simulink model "siasun_config_casadi_VS_lsj_sim_16a"  (R2020a)
(part 10 of 11)

-0.644078158142065,-0.644802838030618,-0.645527980509147,-0.646253539045693,-0.646979466239331,-0.647705713820167,-0.648432232649345,-0.649158972719038,-0.649885883152457,-0.650612912203845,-0.651340007258479,-0.652067114832670,-0.652794180573764,-0.653521149260139,-0.654247964801207,-0.654974570237416,-0.655700907740245,-0.656426918612209,-0.657152543286855,-0.657877721328767,-0.658602391433560,-0.659326491427883,-0.660049958269421,-0.660772728046890,-0.661494735980042,-0.662215916419663,-0.662936202847570,-0.663655527876618,-0.664373823250693,-0.665091019844716,-0.665807047664642,-0.666521835847457,-0.667235312661186,-0.667947405504885,-0.668658040908642,-0.669367144533582,-0.670074641171864,-0.670780454746678,-0.671484508312250,-0.672186724053839,-0.672887023287738,-0.673585326461276,-0.674281553152812,-0.674975622072357,-0.675667451285948,-0.676356959326780,-0.677044065777502,-0.677728691290112,-0.678410757585964,-0.679090187455765,-0.679766904759571,-0.680440834426794,-0.681111902456198,-0.681780035915898,-0.682445162943365,-0.683107212745418,-0.683766115598233,-0.684421802847337,-0.685074206907609,-0.685723261263280,-0.686368900467938,-0.687011060144518,-0.687649676985311,-0.688284688751960,-0.688916034275461,-0.689543653456161,-0.690167487263763,-0.690787477737318,-0.691403567985234,-0.692015702185270,-0.692623825584536,-0.693227884499498,-0.693827826315972,-0.694423599489128,-0.695015153543487,-0.695602439072925,-0.696185407740670,-0.696764012279302,-0.697338206490753,-0.697907945246309,-0.698473184486608,-0.699033881221643,-0.699589993530754,-0.700141480562639,-0.700688302535347,-0.701230420736280,-0.701767797522191,-0.702300396319188,-0.702828181622730,-0.703351118997629,-0.703869175078051,-0.704382317567512,-0.704890515238883,-0.705393737934386,-0.705891956565598,-0.706385143113447,-0.706873270628213,-0.707356313229530,-0.707834246106384,-0.708307045517114,-0.708774688789411,-0.709237154320320,-0.709694421576238,-0.710146471092914,-0.710593284475450,-0.711034844398302,-0.711471134605276,-0.711902139909533,-0.712327846193585,-0.712748240409299,-0.713163310577893,-0.713573045789936,-0.713977436205353,-0.714376473053420,-0.714770148632767,-0.715158456311373,-0.715541390526574,-0.715918946785056,-0.716291121662859,-0.716657912805375,-0.717019318927349,-0.717375339812879,-0.717725976315414,-0.718071230357757,-0.718411104932064,-0.718745604099843,-0.719074732991955,-0.719398497808613,-0.719716905819383,-0.720029965363186,-0.720337685848291,-0.720640077752322,-0.720937152622258,-0.721228923074427,-0.721515402794511,-0.721796606537546,-0.722072550127918,-0.722343250459368,-0.722608725494989,-0.722868994267226,-0.723124076877877,-0.723373994498094,-0.723618769368379,-0.723858424798589,-0.724092985167932,-0.724322475924970,-0.724546923587618,-0.724766355743141,-0.724980801048160,-0.725190289228646,-0.725394851079925,-0.725594518466673,-0.725789324322922,-0.725979302652053,-0.726164488526803,-0.726344918089258,-0.726520628550861,-0.726691658192404,-0.726858046364034,-0.727019833485249,-0.727177061044901,-0.727329771601194,-0.727478008781686,-0.727621817283284,-0.727761242872251,-0.727896332384203,-0.728027133724106,-0.728153695866281,-0.728276068854401,-0.728394303801490,-0.728508452889927,-0.728618569371443,-0.728724707567122,-0.728826922867398,-0.728925271732062,-0.729019811690254,-0.729110601340468,-0.729197700350552,-0.729281169457705,-0.729361070468478,-0.729437466258778,-0.729510420773860,-0.729579999028335,-0.729646267106166,-0.729709292160669,-0.729769142414511,-0.729825887159713,-0.729879596757648,-0.729930342639043,-0.729978197303977,-0.730023234321880,-0.730065528331537,-0.730105155041085,-0.730142191228012,-0.730176714739162,-0.730208804490729,-0.730238540468259,-0.730266003726654,-0.730291276390166,-0.730314441652400,-0.730335583776315,-0.730354788094221,-0.730372141007782,-0.730387729988013,-0.730401643575283,-0.730413971379315,-0.730424804079181,-0.730434233423308,-0.730442352229477,-0.730449254384818,-0.730455034845817,-0.730459789638311,-0.730463615857491,-0.730466611667898,-0.730468876303428,-0.730470510067329,-0.730471614332203,-0.730472291540001,-0.730472645202032,-0.730472779898952,-0.730472801280773];

    kkend = size(traj,2);
    ktime = kkend/1000;
    
    stageTime = 10;
    
    if time<=stageTime
        time=0;
        kk = 1;
    elseif stageTime<time && time<=(stageTime+ktime)
        time=time-stageTime;
        kk = floor(time*1000);
        if(kk == 0)
            kk = 1;
        end
    else
        time = ktime;
        kk = kkend;
    end
    
    initq = traj(:,1);
    q = traj(:,1);
    
    if time>=ktime
        q = traj(:,end);
    elseif time < ktime
        q = traj(:,kk);
    end    
    
end
